simulink model "ControlSimulation"  (R2016b)
settings: Solver=VariableStepAuto  StartTime=0.0  StopTime=10.0  RelTol=1e-3  EnableMultiTasking=on
settings Model: Creator=Guilherme  LastModifiedBy=Guilherme
settings OptimizationCC: LifeSpan=inf
settings DebuggingCC: SFUnexpectedBacktrackingDiag=warning  SFNoUnconditionalDefaultTransitionDiag=warning  SFExecutionAtInitializationDiag=none
settings GRTTargetCC: TargetLangStandard=C89/C90 (ANSI)  GeneratePreprocessorConditionals=Disable all
settings ConfigComp: CovMetricSettings=dw  CovHtmlReporting=on  CovSaveCumulativeToWorkspaceVar=on  CovSaveSingleToWorkspaceVar=on  CovExternalEMLEnable=off

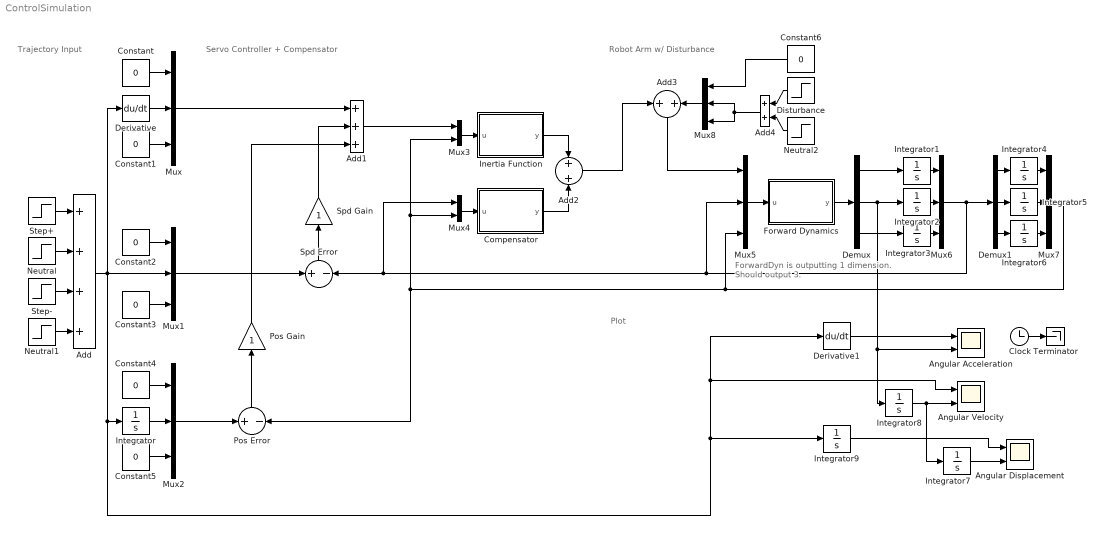
== system ControlSimulation ==
  note: ForwardDyn is outputting 1 dimension.
      | Should output 3.
  note: Plot
  note: Robot Arm w/ Disturbance
  note: Servo Controller + Compensator
  note: Trajectory Input
  Add : Sum  Inputs=++++
  Add1 : Sum  Inputs=+++
  Add2 : Sum
  Add3 : Sum
  Add4 : Sum
  Angular Acceleration : Scope  NumInputPorts=2
  Angular Displacement : Scope  NumInputPorts=2
  Angular Velocity : Scope  NumInputPorts=2
  Clock : Clock
  Compensator : MATLAB Function  TreatAsAtomicUnit=on
  Constant{,1..6} (7 alike) : Constant  Value=0
  Demux : Demux  Outputs=3
  Demux1 : Demux  Outputs=3
  Derivative : Derivative
  Derivative1 : Derivative
  Disturbance : Step  Time=3  SampleTime=0
  Forward Dynamics : MATLAB Function  TreatAsAtomicUnit=on
  Inertia Function : MATLAB Function  TreatAsAtomicUnit=on
  Integrator{,1..9} (10 alike) : Integrator
  Mux{,1..2,5..8} (7 alike) : Mux  Inputs=3
  Mux3 : Mux  Inputs=2
  Mux4 : Mux  Inputs=2
  Neutral : Step  Time=2  After=-1.5  SampleTime=0
  Neutral1 : Step  Time=7  After=1.5  SampleTime=0
  Neutral2 : Step  Time=8  After=-1  SampleTime=0
  Pos Error : Sum  Inputs=+-
  Pos Gain : Gain
  Spd Error : Sum  Inputs=+-
  Spd Gain : Gain
  Step+ : Step  Time=0  After=1.5  SampleTime=0
  Step- : Step  Time=5  After=-1.5  SampleTime=0
  Terminator : Terminator
  wires:
  Step+/1 -> Add/1
  Neutral/1 -> Add/2
  Step-/1 -> Add/3
  Neutral1/1 -> Add/4
  Add/1 -> Mux1/2, Integrator/1, Angular Velocity/1, Derivative1/1, Integrator9/1, Derivative/1
  Constant4/1 -> Mux2/1
  Integrator/1 -> Mux2/2
  Constant5/1 -> Mux2/3
  Constant1/1 -> Mux/3
  Constant/1 -> Mux/1
  Derivative/1 -> Mux/2
  Constant2/1 -> Mux1/1
  Constant3/1 -> Mux1/3
  Mux2/1 -> Pos Error/1
  Mux1/1 -> Spd Error/1
  Spd Error/1 -> Spd Gain/1
  Pos Error/1 -> Pos Gain/1
  Spd Gain/1 -> Add1/2
  Pos Gain/1 -> Add1/3
  Mux/1 -> Add1/1
  Mux3/1 -> Inertia Function/1(u)
  Add1/1 -> Mux3/1
  Mux4/1 -> Compensator/1(u)
  Inertia Function/1(y) -> Add2/1
  Compensator/1(y) -> Add2/2
  Mux5/1 -> Forward Dynamics/1(u)
  Add3/1 -> Mux5/1
  Forward Dynamics/1(y) -> Demux/1
  Demux/1 -> Integrator1/1
  Demux/2 -> Integrator8/1, Angular Acceleration/2, Integrator2/1
  Demux/3 -> Integrator3/1
  Integrator1/1 -> Mux6/1
  Integrator2/1 -> Mux6/2
  Integrator3/1 -> Mux6/3
  Demux1/1 -> Integrator4/1
  Demux1/2 -> Integrator5/1
  Demux1/3 -> Integrator6/1
  Integrator4/1 -> Mux7/1
  Integrator5/1 -> Mux7/2
  Integrator6/1 -> Mux7/3
  Mux6/1 -> Demux1/1, Mux4/1, Spd Error/2, Mux5/2
  Mux7/1 -> Mux5/3, Pos Error/2, Mux4/2, Mux3/2
  Clock/1 -> Terminator/1
  Integrator8/1 -> Integrator7/1, Angular Velocity/2
  Integrator9/1 -> Angular Displacement/1
  Integrator7/1 -> Angular Displacement/2
  Derivative1/1 -> Angular Acceleration/1
  Disturbance/1 -> Add4/1
  Neutral2/1 -> Add4/2
  Mux8/1 -> Add3/2
  Constant6/1 -> Mux8/1
  Add4/1 -> Mux8/2, Mux8/3
  Add2/1 -> Add3/1

== matlab function ControlSimulation/Compensator ==
  data: u input; y output
function y = fcn(u)

y = Compensator([u(1); u(2); u(3); u(4); u(5); u(6)]);

== matlab function ControlSimulation/Inertia Function ==
  data: u input; y output
function y = fcn(u)

y = InertiaFunc([u(1); u(2); u(3); u(4); u(5); u(6)]);

== matlab function ControlSimulation/Forward Dynamics ==
  data: u input; y output
function y = fcn(u)

y = ForwardDyn_Ctrl([u(1); u(2); u(3); u(4); u(5); u(6); u(7); u(8); u(9)]);
